simulink model "Verifica_LQR_06072026"  (R2025b)
settings: Solver=VariableStepAuto  StartTime=0.0  StopTime=10.0  RelTol=1e-3
undefined symbols (not defined in the file): A, B, K_LQR_i, K_LQR_x, m, n, r
settings Model: Creator=salvo  LastModifiedBy=salvo

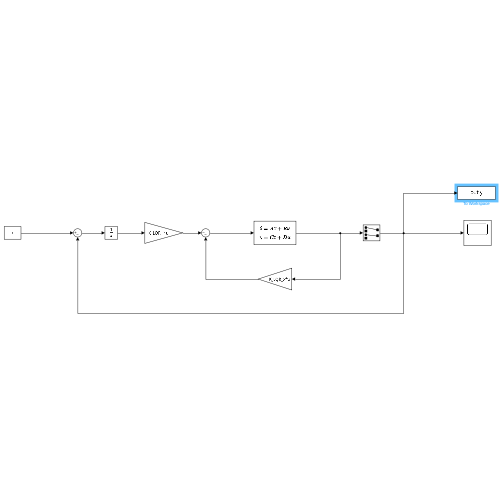
[thumbnail: Simulink's stored preview of the top-level diagram]
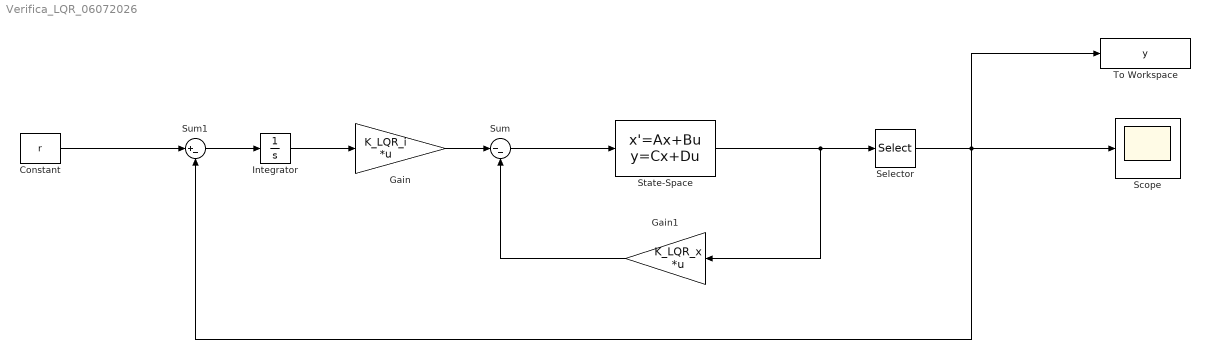
== system Verifica_LQR_06072026 ==
  Constant : Constant  Value=r
  Gain : Gain  Gain=K_LQR_i  Multiplication=Matrix(K*u)
  Gain1 : Gain  Gain=K_LQR_x  Multiplication=Matrix(K*u)
  Integrator : Integrator
  Scope : Scope
      settings: ActiveDisplayYMinimum=-0.13750000000000023  ActiveDisplayYMaximum=0.23750000000000027
  Selector : Selector  InputPortWidth=4  IndexOptions=Index vector (dialog)  Indices=[1 3]  OutputSizes=1
  State-Space : StateSpace  A=A  B=B  C=eye(n)  D=zeros(n,m)  InitialCondition=0
  Sum : Sum  Inputs=|--
  Sum1 : Sum  Inputs=|+-
  To Workspace : ToWorkspace  VariableName=y  SaveFormat=Timeseries  SampleTime=-1
  wires:
  Constant/1 -> Sum1/1
  Sum1/1 -> Integrator/1
  Integrator/1 -> Gain/1
  Gain/1 -> Sum/1
  Gain1/1 -> Sum/2
  Sum/1 -> State-Space/1
  State-Space/1 -> Selector/1, Gain1/1
  Selector/1 -> To Workspace/1, Sum1/2, Scope/1
